simulink model "PenduloMuelle"  (R2024b)
settings: Solver=FixedStepAuto  StartTime=0.0  StopTime=10.0  FixedStep=0.01  RelTol=1e-3
model workspace (MATLAB code in the model file):
  | k = 40;
  | m = 0.25;
  | L = 0.5 + 0.02*randn(1,5);
undefined symbols (not defined in the file): g
settings Model: Creator=Miguel  LastModifiedBy=Miguel

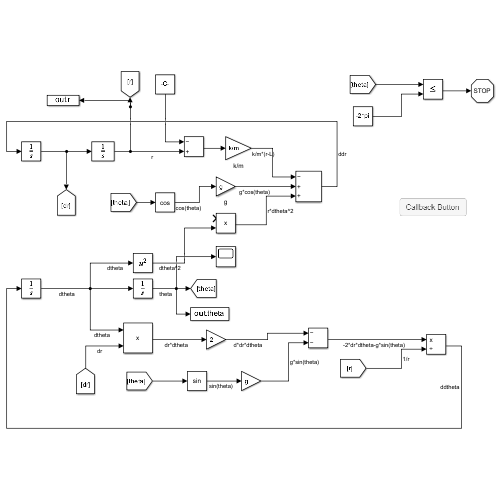
[thumbnail: Simulink's stored preview of the top-level diagram]
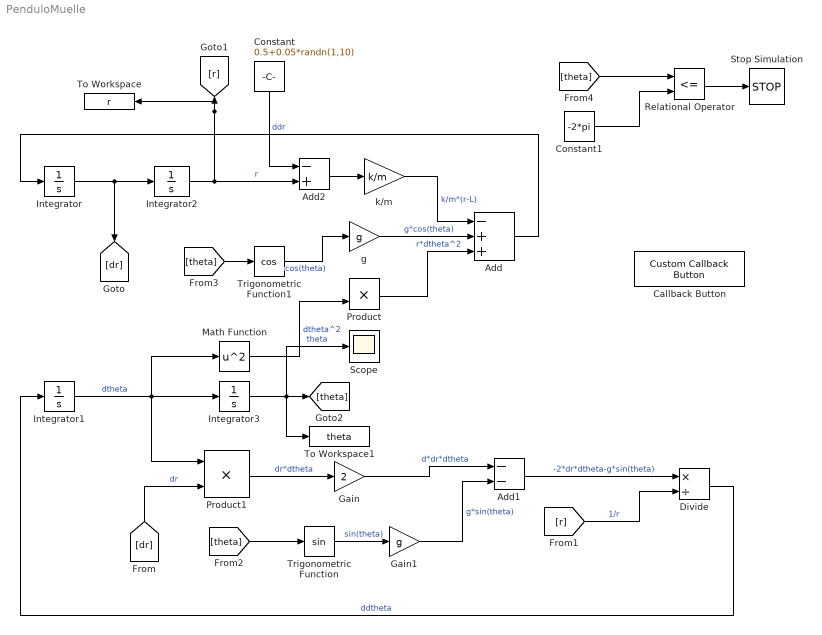
== system PenduloMuelle ==
  Add : Sum  Inputs=-++
  Add1 : Sum  Inputs=--
  Add2 : Sum  Inputs=-+
  Callback Button : CustomCallbackButton  Configuration="{\"components\":[{\"name\":\"BackgroundImageComponent\",\"settings\":{\"image\":{\"size\":[0,0],\"src\":\"default\",\"srcOrientation\":\"Right\"},\"position\":[0,0,1,1]}},{\"name\":\"ButtonStateComponent\",\"settings\":{\"buttonType\":\"momentary\",\"clickFcn\":\"r = out.r;\\ntheta = out.theta;\\nt = out.tout;\\n\\nfigure\\nplot(t,r,'b','linewidth',2)\\ngrid on\\nxlabel('Tiempo (s)')\\nylabel('r (m)')\\n\\nfigure\\nplot(t,theta,'LineWidth',2)\\ngrid on\\nxlabel('Tiempo (s)')\\nylabel('\\\\theta (rad)')\",\"onValue\":1,\"position\":[0,0,1,1],\"pressDelay\":\"500\",\"pressFcn\":\"\",\"repeatInterval\":\"0\",\"states\":[{\"horizontalAlignment\":\"center\",\"image\":{\"position\":[0,0,1,1],\"size\":[1,1],\"src\":\"default\",\"srcOrientation\":\"Right\"},\"label\":{\"color\":[0.01176470588,0.01176470588,0.01176470588,1],\"icon\":{\"size\":[0,0],\"src\":\"default\",\"srcOrientation\":\"Right\"},\"iconOffset\":0,\"iconPlacement\":\"left\",\"opacity\":1,\"show\":true,\"text\":{\"content\":\"Callback Button\",\"font\":\"Helvetica\"}},\"labelOffset\":[0,0],\"verticalAlignment\":\"middle\"},{\"horizontalAlignment\":\"center\",\"image\":{\"position\":[0,0,1,1],\"size\":[1,1],\"src\":\"default\",\"srcOrientation\":\"Right\"},\"label\":{\"color\":[0.01176470588,0.01176470588,0.01176470588,1],\"icon\":{\"size\":[0,0],\"src\":\"default\",\"srcOrientation\":\"Right\"},\"iconOffset\":0,\"iconPlacement\":\"left\",\"opacity\":1,\"show\":true,\"text\":{\"content\":\"Callback Button\",\"font\":\"Helvetica\"}},\"labelOffset\":[0,0],\"verticalAlignment\":\"middle\"},{\"horizontalAlignment\":\"center\",\"image\":{\"position\":[0,0,1,1],\"size\":[1,1],\"src\":\"default\",\"srcOrientation\":\"Right\"},\"label\":{\"color\":[0.01176470588,0.01176470588,0.01176470588,1],\"icon\":{\"size\":[0,0],\"src\":\"default\",\"srcOrientation\":\"Right\"},\"iconOffset\":0,\"iconPlacement\":\"left\",\"opacity\":1,\"show\":true,\"text\":{\"content\":\"Callback Button\",\"font\":\"Helvetica\"}},\"labelOffset\":[0,0],\"verticalAlignment\":\"middle\"},{\"horizontalAlignment\":\"center\",\"image\":{\"position\":[0,0,1,1],\"size\":[1,1],\"src\":\"default\",\"srcOrientation\":\"Right\"},\"label\":{\"color\":[0.01176470588,0.01176470588,0.01176470588,1],\"icon\":{\"size\":[0,0],\"src\":\"default\",\"srcOrientation\":\"Right\"},\"iconOffset\":0,\"iconPlacement\":\"left\",\"opacity\":1,\"show\":true,\"text\":{\"content\":\"Callback Button\",\"font\":\"Helvetica\"}},\"labelOffset\":[0,0],\"verticalAlignment\":\"middle\"}]}},{\"name\":\"ForegroundImageComponent\",\"settings\":{\"image\":{\"size\":[0,0],\"src\":\"default\",\"srcOrientation\":\"Right\"},\"isForeground\":1,\"position\":[0,0,1,1]}}],\"settings\":{\"BindingType\":\"standalone\",\"backgroundColor\":[244,244,244,1],\"backgroundOffset\":0.2,\"backgroundOpacity\":1,\"fixedAspectRatio\":\"off\",\"foregroundColor\":[0.01176470588,0.01176470588,0.01176470588,1],\"migratedFromLegacy\":true,\"useBackgroundColor\":true,\"variant\":\"callback\",\"version\":\"R2023a\"},\"type\":\"Button\"}"  CustomBackgroundColor="{\"color\":[0.9568627451,0.9568627451,0.9568627451],\"show\":true}"
  Constant : Constant  Value=0.5+0.05*randn(1,10)
  Constant1 : Constant  Value=-2*pi
  Divide : Product  Inputs=*/
  Gain : Gain  Gain=2
  Gain1 : Gain  Gain=g
  Integrator : Integrator  InitialCondition=-0.5
  Integrator1 : Integrator
  Integrator2 : Integrator  InitialCondition=L
  Integrator3 : Integrator  InitialCondition=(60*pi/180)
  Math Function : Math  Operator=square
  Product : Product
  Product1 : Product
  Relational Operator : RelationalOperator  Operator=<=  OutDataTypeStr=boolean  RndMeth=Simplest  InputSameDT=off
  Scope : Scope
  Stop Simulation : Stop
  To Workspace : ToWorkspace  VariableName=r  SampleTime=-1
  To Workspace1 : ToWorkspace  VariableName=theta  SampleTime=-1
  Trigonometric Function : Trigonometry
  Trigonometric Function1 : Trigonometry  Operator=cos
  g : Gain  Gain=g
  k/m : Gain  Gain=k/m
  wires:
  Integrator1/1 -> Integrator3/1, Product1/1, Math Function/1  "dtheta"
  Math Function/1 -> Product/2  "dtheta^2"
  Product/1 -> Add/3  "r*dtheta^2"
  k/m/1 -> Add/1  "k/m*(r-L)"
  Add/1 -> Integrator/1  "ddr"
  Integrator/1 -> [dr], Integrator2/1
  [dr] -> Product1/2  "dr"
  Product1/1 -> Gain/1  "dr*dtheta"
  Gain/1 -> Add1/1  "d*dr*dtheta"
  Add1/1 -> Divide/1  "-2*dr*dtheta-g*sin(theta)"
  Integrator2/1 -> Add2/2, To Workspace/1, [r]  "r"
  [r] -> Divide/2  "1/r"
  Divide/1 -> Integrator1/1  "ddtheta"
  Integrator3/1 -> Scope/1, To Workspace1/1, [theta]  "theta"
  [theta] -> Trigonometric Function/1
  Trigonometric Function/1 -> Gain1/1  "sin(theta)"
  Gain1/1 -> Add1/2  "g*sin(theta)"
  [theta] -> Trigonometric Function1/1
  Trigonometric Function1/1 -> g/1  "cos(theta)"
  g/1 -> Add/2  "g*cos(theta)"
  Add2/1 -> k/m/1
  Constant/1 -> Add2/1
  [theta] -> Relational Operator/1
  Constant1/1 -> Relational Operator/2
  Relational Operator/1 -> Stop Simulation/1
